simulink model "Hopper_ground"  (Simulink 7.9)
settings: Solver=ode45  StartTime=0.0  StopTime=100  MaxStep=1e-2  RelTol=1e-6
values from neighbouring files (symbols this model uses):
  Amp = coeff(1)    [SSheight3.m]    (also in SimParam_cpg.m = 0.0249; TwoD_search.m = AMP(jj,1); linear_search.m = leg_length/4)
undefined symbols (not defined in the file or in its folder): b_damper, Freq, k_spring, m_mass
libraries: simulink x1
settings Model: Creator=Metti  LastModifiedBy=Metti
settings SolverCC: ZeroCrossControl=DisableAll

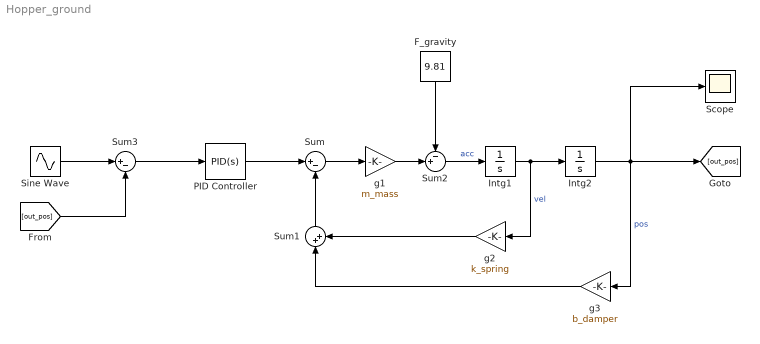
== system Hopper_ground ==
  F_gravity : Constant  Value=9.81
  Intg1 : Integrator
  Intg2 : Integrator
  PID Controller : simulink/Continuous/PID Controller  Controller=PID  TimeDomain=Continuous-time  SampleTime=1  IntegratorMethod=Forward Euler  FilterMethod=Forward Euler  Form=Parallel  P=3964.11703351066  I=6337.67154775249  D=213.34057643197  N=428.843364138649  InitialConditionSource=internal  InitialConditionForIntegrator=0  InitialConditionForFilter=0  ExternalReset=none  LimitOutput=off  UpperSaturationLimit=inf  LowerSaturationLimit=-inf  LinearizeAsGain=off  AntiWindupMode=none  Kb=1  TrackingMode=off  Kt=1  PParamMin=[]  PParamMax=[]  IParamMin=[]  IParamMax=[]  DParamMin=[]  DParamMax=[]  NParamMin=[]  NParamMax=[]  KbParamMin=[]  KbParamMax=[]  KtParamMin=[]  KtParamMax=[]  POutMin=[]  POutMax=[]  IOutMin=[]  IOutMax=[]  DOutMin=[]  DOutMax=[]  NOutMin=[]  NOutMax=[]  KbOutMin=[]  KbOutMax=[]  KtOutMin=[]  KtOutMax=[]  IntegratorOutMin=[]  IntegratorOutMax=[]  FilterOutMin=[]  FilterOutMax=[]  SumOutMin=[]  SumOutMax=[]  SumI1OutMin=[]  SumI1OutMax=[]  SumI2OutMin=[]  SumI2OutMax=[]  SumI3OutMin=[]  SumI3OutMax=[]  SumDOutMin=[]  SumDOutMax=[]  SaturationOutMin=[]  SaturationOutMax=[]  IntegratorContinuousStateAttributes=''  IntegratorStateMustResolveToSignalObject=off  IntegratorRTWStateStorageClass=Auto  FilterContinuousStateAttributes=''  FilterStateMustResolveToSignalObject=off  FilterRTWStateStorageClass=Auto
  Scope : Scope
  Sine Wave : Sin  Amplitude=Amp  Frequency=Freq  SampleTime=0
  Sum : Sum  Inputs=|+-
  Sum1 : Sum  Inputs=|++
  Sum2 : Sum  Inputs=-+|
  Sum3 : Sum  Inputs=|+-
  g1 : Gain  Gain=m_mass
  g2 : Gain  Gain=k_spring
  g3 : Gain  Gain=b_damper
  wires:
  Intg1/1 -> g2/1, Intg2/1  "vel"
  Intg2/1 -> g3/1, [out_pos], Scope/1  "pos"
  g3/1 -> Sum1/1
  g2/1 -> Sum1/2
  Sum1/1 -> Sum/2
  Sum/1 -> g1/1
  PID Controller/1 -> Sum/1
  g1/1 -> Sum2/2
  Sum2/1 -> Intg1/1  "acc"
  F_gravity/1 -> Sum2/1
  Sine Wave/1 -> Sum3/1
  Sum3/1 -> PID Controller/1
  [out_pos] -> Sum3/2
